simulink model "control_system_nl_lin_ref"  (R2025b)
settings: Solver=FixedStepAuto  StartTime=0.0  StopTime=20  FixedStep=0.01  RelTol=1e-3
values from neighbouring files (symbols this model uses):
  A1 = 0    [init_control_system_nl_lin_ref.m]
  A2 = 0    [init_control_system_nl_lin_ref.m]
  K = K_aug(1:end-1)    [init_control_system_nl_lin_ref.m]
  k = 15    [init_control_system_nl_lin_ref.m]
  ki = K_aug(end)    [init_control_system_nl_lin_ref.m]
  x0 = [1 1.5]'    [init_control_system_nl_lin_ref.m]
  xeq = P2    [init_control_system_nl_lin_ref.m]
  yd = xeq.x1    [init_control_system_nl_lin_ref.m]
libraries: simulink x1
settings Model: Creator=ricca  LastModifiedBy=ricca

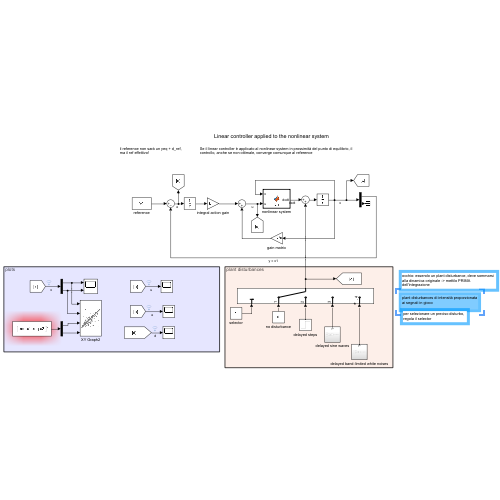
[thumbnail: Simulink's stored preview of the top-level diagram]
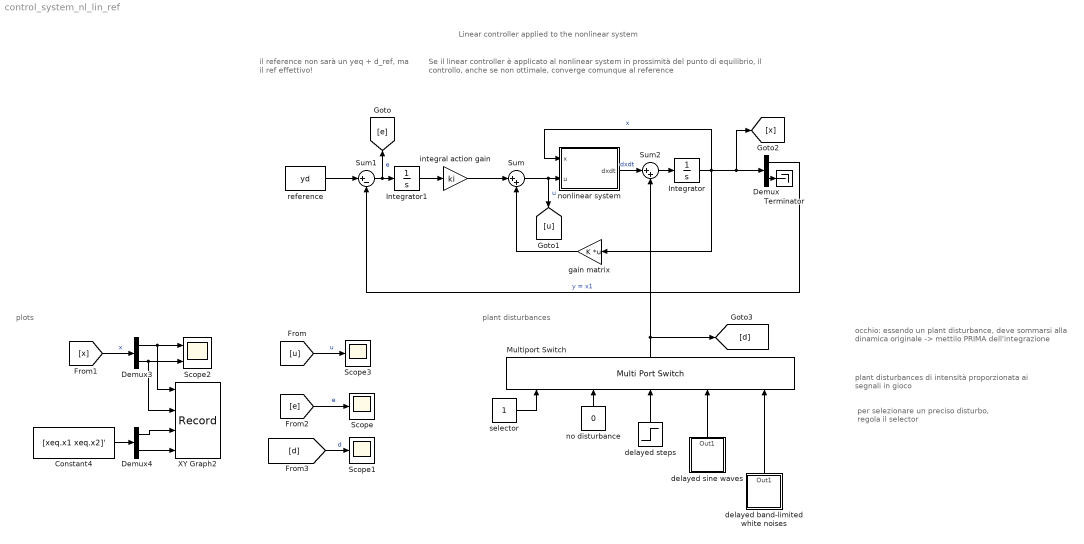
== system control_system_nl_lin_ref ==
  note: plant disturbances
  note: Linear controller applied to the nonlinear system
  note: Se il linear controller è applicato al nonlinear system in prossimità del punto di equilibrio, il controllo, anche se non ottimale, converge comunque al reference
  note: il reference non sarà un yeq + d_ref, ma il ref effettivo!
  note: plots
  note: occhio: essendo un plant disturbance, deve sommarsi alla dinamica originale -> mettilo PRIMA dell'integrazione
  note: per selezionare un preciso disturbo, regola il selector
  note: plant disturbances di intensità proporzionata ai segnali in gioco
  Constant4 : Constant  Value=[xeq.x1 xeq.x2]'
  Demux : Demux  Outputs=2
  Demux3 : Demux  Outputs=2
  Demux4 : Demux  Outputs=2
  Integrator : Integrator  InitialCondition=[x0(1), x0(2)]'
  Integrator1 : Integrator
  Multiport Switch : MultiPortSwitch  Inputs=4  SaturateOnIntegerOverflow=off  InputSameDT=off
  Scope : Scope
      settings: ActiveDisplayYMinimum=-1  ActiveDisplayYMaximum=1
  Scope1 : Scope
      settings: ActiveDisplayYMinimum=-0.074999999999999983  ActiveDisplayYMaximum=0.67499999999999993
  Scope2 : Scope  NumInputPorts=2
      settings: ActiveDisplayYMinimum=0.66452669290968613  ActiveDisplayYMaximum=4.0192597638128262  DataLoggingVariableName=ScopeData2
  Scope3 : Scope
      settings: ActiveDisplayYMinimum=-1  ActiveDisplayYMaximum=1  DataLoggingVariableName=ScopeData3
  Sum : Sum  Inputs=|++
  Sum1 : Sum  Inputs=|+-
  Sum2 : Sum  Inputs=|++
  Terminator : Terminator
  XY Graph2 : Record  NumPorts=4.0  FileSettingsInternal="{\"entries\":[{\"content\":{\"excelSettings\":{\"content\":{},\"type\":\"Streamout.ExcelSettings\"},\"parquetSettings\":{\"content\":{},\"type\":\"Streamout.ParquetSettings\"}},\"type\":\"Streamout.FileSettingStorage\",\"uuid\":\"\"}],\"packageUris\":[\"http:\\/\\/schema.mathworks.com\\/mf0\\/streamout_blocks\\/R2020a\"],\"version\":\"1.0\"}"  FrameSettings=[0, 0, 0, 0]  Layout=[1 1]  SignalsInternal="{\"entries\":[{\"content\":{\"signals\":[{\"content\":{\"blockPath\":[],\"dimensions\":[1],\"domain\":\"\",\"lineColor\":\"#139fff\",\"plots\":[ 1 ],\"port\":1,\"signalID\":1,\"signalName\":\"Demux3:1\"},\"type\":\"RecordBlkView.Signal\",\"uuid\":\"\"},{\"content\":{\"blockPath\":[],\"dimensions\":[1],\"domain\":\"\",\"lineColor\":\"#139fff\",\"plots\":[ 1 ],\"port\":2,\"signalID\":2,\"signalName\":\"Demux3:2\"},\"type\":\"RecordBlkView.Signal\",\"uuid\":\"\"},{\"content\":{\"blockPath\":[],\"dimensions\":[1],\"domain\":\"\",\"lineColor\":\"#a2142f\",\"lineWidth\":20,\"plots\":[ 1 ],\"port\":3,\"signalID\":3,\"signalName\":\"Demux4:1\"},\"type\":\"RecordBlkView.Signal\",\"uuid\":\"\"},{\"content\":{\"blockPath\":[],\"dimensions\":[1],\"domain\":\"\",\"lineColor\":\"#a2142f\",\"lineWidth\":20,\"plots\":[ 1 ],\"port\":4,\"signalID\":4,\"signalName\":\"Demux4:2\"},\"type\":\"RecordBlkView.Signal\",\"uuid\":\"\"}]},\"type\":\"RecordBlkView.InputSignals\",\"uuid\":\"\"}],\"packageUris\":[\"http:\\/\\/schema.mathworks.com\\/mf0\\/streamout_blocks\\/R2020a\"],\"version\":\"1.0\"}"  VisualizationBindings="{\"xyplotplugin\":{\"info\":[{\"series\":[{\"bindingParametersList\":[{\"parameter\":\"X-Axis\",\"signalID\":3,\"signalName\":\"Demux4:1\"},{\"parameter\":\"Y-Axis\",\"signalID\":4,\"signalName\":\"Demux4:2\"}],\"seriesID\":0},{\"bindingParametersList\":[{\"parameter\":\"X-Axis\",\"signalID\":1,\"signalName\":\"Demux3:1\"},{\"parameter\":\"Y-Axis\",\"signalID\":2,\"signalName\":\"Demux3:2\"}],\"seriesID\":1}],\"subplotID\":1}]}}"  CompatibilityTag=XY
  delayed band-limited white noises : Subsystem
  delayed sine waves : Subsystem
  delayed steps : Step  Time=[7 8]'  After=[0.5 0.6]'  SampleTime=0
  gain matrix : Gain  Gain=K  Multiplication=Matrix(K*u)
  integral action gain : Gain  Gain=ki
  no disturbance : Constant  Value=0  OutDataTypeStr=Inherit: Inherit via back propagation
  nonlinear system : MATLAB Function  TreatAsAtomicUnit=on
  reference : Constant  Value=yd
  selector : Constant
  wires:
  gain matrix/1 -> Sum/2
  Demux/1 -> Sum1/2  "y = x1"
  Integrator/1 -> [x], Demux/1, gain matrix/1, nonlinear system/1(x)  "x"
  integral action gain/1 -> Sum/1
  Integrator1/1 -> integral action gain/1
  Sum1/1 -> [e], Integrator1/1  "e"
  reference/1 -> Sum1/1
  Demux/2 -> Terminator/1
  Demux4/1 -> XY Graph2/3
  Demux4/2 -> XY Graph2/4
  Demux3/1 -> XY Graph2/1, Scope2/1
  Constant4/1 -> Demux4/1
  [x] -> Demux3/1  "x"
  [u] -> Scope3/1  "u"
  Demux3/2 -> XY Graph2/2, Scope2/2
  Multiport Switch/1 -> [d], Sum2/2
  [e] -> Scope/1  "e"
  [d] -> Scope1/1  "d"
  delayed sine waves/1(Out1) -> Multiport Switch/4
  delayed band-limited white noises/1(Out1) -> Multiport Switch/5
  delayed steps/1 -> Multiport Switch/3
  selector/1 -> Multiport Switch/1
  no disturbance/1 -> Multiport Switch/2
  Sum/1 -> [u], nonlinear system/2(u)  "u"
  nonlinear system/1(dxdt) -> Sum2/1  "dxdt"
  Sum2/1 -> Integrator/1

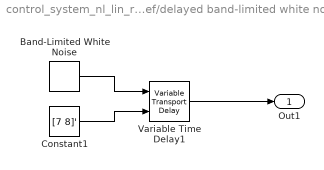
== system control_system_nl_lin_ref/delayed band-limited white noises ==
  Band-Limited White Noise : simulink/Sources/Band-Limited White Noise  Cov=[0.01 0.01]'  Ts=0.1  seed=[23341 23342]'
  Constant1 : Constant  Value=[7 8]'
  Variable Time Delay1 : VariableTransportDelay  MaximumDelay=10
  Out1 : Outport
  wires:
  Constant1/1 -> Variable Time Delay1/2
  Band-Limited White Noise/1 -> Variable Time Delay1/1
  Variable Time Delay1/1 -> Out1/1

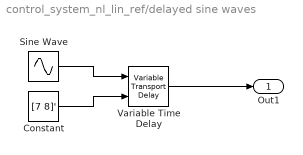
== system control_system_nl_lin_ref/delayed sine waves ==
  Constant : Constant  Value=[7 8]'
  Sine Wave : Sin  Amplitude=[0.5 0.6]'  Bias=[0 0]'  SampleTime=0
  Variable Time Delay : VariableTransportDelay  MaximumDelay=10
  Out1 : Outport
  wires:
  Sine Wave/1 -> Variable Time Delay/1
  Variable Time Delay/1 -> Out1/1
  Constant/1 -> Variable Time Delay/2

== matlab function control_system_nl_lin_ref/nonlinear system ==
  data: x input; u input; dxdt output; A1 parameter; A2 parameter; k parameter
function dxdt = fcn(x,u,A1, A2, k)

dxdt = [-x(1) + A2 + k*x(2)*exp(-x(2));           
        -x(2) + A1 + k*x(1)*exp(-x(1)) + u];    

%% se vuoi testare la sensibilità rispetto a unmodelled dynamics  Delta_f, uncommmenta i Delta_f e dxdt sotto, e commmenta il dxdt sopra. Ricordati di aumentare k_law, come da teoria!

% Delta_f = 0.2*sin(x(1));
% dxdt = [-x(1) + A2 + k*x(2)*exp(-x(2)) + Delta_f;           
%         -x(2) + A1 + k*x(1)*exp(-x(1)) + Delta_f + u];    

%% se vuoi testare la sensibilità rispetto a parametric uncertainties del 10% su k, uncommmenta dxdt sotto, e commmenta il dxdt sopra.

% dxdt = [-x(1) + A2 + (k+0.10*k)*x(2)*exp(-x(2));           
%         -x(2) + A1 + (k+0.10*k)*x(1)*exp(-x(1)) + u];   

end
